simulink model "pkadai11"  (R2021b)
settings: Solver=VariableStepAuto  StartTime=0.0  StopTime=100  RelTol=1e-3
settings Model: Creator=is221042  LastModifiedBy=is221042

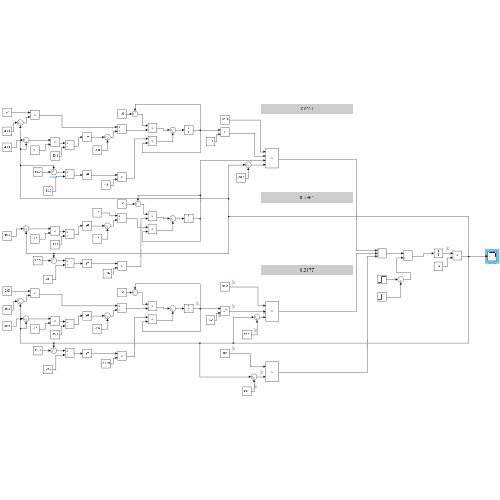
[thumbnail: Simulink's stored preview of the top-level diagram]
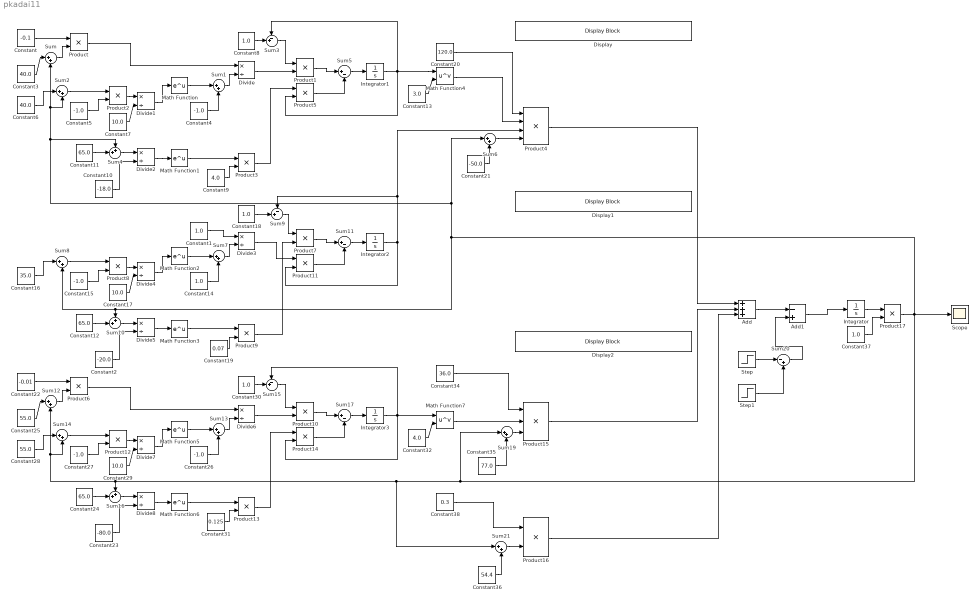
== system pkadai11 ==
  Add : Sum  Inputs=+++
  Add1 : Sum  Inputs=-+
  Constant : Constant  Value=-0.1
  Constant{1,8,14,18,30,37} (6 alike) : Constant  Value=1.0
  Constant10 : Constant  Value=-18.0
  Constant11 : Constant  Value=65.0
  Constant12 : Constant  Value=65.0
  Constant13 : Constant  Value=3.0
  Constant{4..5,15,26..27} (5 alike) : Constant  Value=-1.0
  Constant16 : Constant  Value=35.0
  Constant17 : Constant  Value=10.0
  Constant19 : Constant  Value=0.07
  Constant2 : Constant  Value=-20.0
  Constant20 : Constant  Value=120.0
  Constant21 : Constant  Value=-50.0
  Constant22 : Constant  Value=-0.01
  Constant23 : Constant  Value=-80.0
  Constant24 : Constant  Value=65.0
  Constant25 : Constant  Value=55.0
  Constant28 : Constant  Value=55.0
  Constant29 : Constant  Value=10.0
  Constant3 : Constant  Value=40.0
  Constant31 : Constant  Value=0.125
  Constant32 : Constant  Value=4.0
  Constant34 : Constant  Value=36.0
  Constant35 : Constant  Value=77.0
  Constant36 : Constant  Value=54.4
  Constant38 : Constant  Value=0.3
  Constant6 : Constant  Value=40.0
  Constant7 : Constant  Value=10.0
  Constant9 : Constant  Value=4.0
  Display : DisplayBlock  LabelPosition=Hide  Format=short  Transparency=1
  Display1 : DisplayBlock  LabelPosition=Hide  Format=short  Transparency=1
  Display2 : DisplayBlock  LabelPosition=Hide  Format=short  Transparency=1
  Divide{,1..8} (9 alike) : Product  Inputs=*/
  Integrator : Integrator  InitialCondition=-65.0
  Integrator1 : Integrator  InitialCondition=0.0529
  Integrator2 : Integrator  InitialCondition=0.4119
  Integrator3 : Integrator  InitialCondition=0.2668
  Math Function{,1..3,5..6} (6 alike) : Math  SaturateOnIntegerOverflow=on
  Math Function4 : Math  Operator=pow  SaturateOnIntegerOverflow=on
  Math Function7 : Math  Operator=pow  SaturateOnIntegerOverflow=on
  Product{,1..3,5..14,16..17} (16 alike) : Product
  Product15 : Product  Inputs=3
  Product4 : Product  Inputs=4
  Scope : Scope
  Step : Step  Time=4  After=5  SampleTime=0
  Step1 : Step  Time=2  After=5  SampleTime=0
  Sum{,1..2,6..8,12..14,19,21} (11 alike) : Sum  Inputs=|++
  Sum10 : Sum  Inputs=++|
  Sum11 : Sum  Inputs=|+-
  Sum15 : Sum  Inputs=-+|
  Sum16 : Sum  Inputs=++|
  Sum17 : Sum  Inputs=|+-
  Sum20 : Sum  Inputs=|-+
  Sum3 : Sum  Inputs=-+|
  Sum4 : Sum  Inputs=++|
  Sum5 : Sum  Inputs=|+-
  Sum9 : Sum  Inputs=-+|
  wires:
  Constant/1 -> Product/1
  Sum/1 -> Product/2
  Constant3/1 -> Sum/1
  Product/1 -> Divide/1
  Math Function/1 -> Sum1/1
  Sum1/1 -> Divide/2
  Constant4/1 -> Sum1/2
  Divide1/1 -> Math Function/1
  Sum2/1 -> Product2/1
  Product2/1 -> Divide1/1
  Constant5/1 -> Product2/2
  Constant6/1 -> Sum2/1
  Constant7/1 -> Divide1/2
  Constant8/1 -> Sum3/2
  Sum3/1 -> Product1/1
  Divide/1 -> Product1/2
  Sum4/1 -> Divide2/1
  Constant10/1 -> Divide2/2
  Constant11/1 -> Sum4/2
  Divide2/1 -> Math Function1/1
  Math Function1/1 -> Product3/1
  Constant9/1 -> Product3/2
  Integrator1/1 -> Product5/2, Math Function4/1, Sum3/1
  Product1/1 -> Sum5/1
  Product3/1 -> Product5/1
  Product5/1 -> Sum5/2
  Sum5/1 -> Integrator1/1
  Constant19/1 -> Product9/2
  Product11/1 -> Sum11/2
  Sum11/1 -> Integrator2/1
  Product7/1 -> Sum11/1
  Divide5/1 -> Math Function3/1
  Constant12/1 -> Sum10/2
  Math Function3/1 -> Product9/1
  Sum7/1 -> Divide3/2
  Constant15/1 -> Product8/2
  Constant17/1 -> Divide4/2
  Integrator2/1 -> Sum9/1, Product4/3, Product11/2
  Constant16/1 -> Sum8/1
  Constant18/1 -> Sum9/2
  Product8/1 -> Divide4/1
  Sum8/1 -> Product8/1
  Math Function2/1 -> Sum7/1
  Constant2/1 -> Divide5/2
  Sum10/1 -> Divide5/1
  Constant14/1 -> Sum7/2
  Sum9/1 -> Product7/1
  Divide4/1 -> Math Function2/1
  Constant1/1 -> Divide3/1
  Divide3/1 -> Product11/1
  Product9/1 -> Product7/2
  Constant13/1 -> Math Function4/2
  Constant20/1 -> Product4/1
  Math Function4/1 -> Product4/2
  Sum6/1 -> Product4/4
  Constant21/1 -> Sum6/2
  Product13/1 -> Product14/1
  Constant31/1 -> Product13/2
  Product14/1 -> Sum17/2
  Sum17/1 -> Integrator3/1
  Product10/1 -> Sum17/1
  Integrator3/1 -> Math Function7/1, Sum15/1, Product14/2
  Divide8/1 -> Math Function6/1
  Constant22/1 -> Product6/1
  Constant24/1 -> Sum16/2
  Constant25/1 -> Sum12/1
  Math Function6/1 -> Product13/1
  Sum13/1 -> Divide6/2
  Constant27/1 -> Product12/2
  Constant29/1 -> Divide7/2
  Product6/1 -> Divide6/1
  Divide6/1 -> Product10/2
  Constant28/1 -> Sum14/1
  Constant30/1 -> Sum15/2
  Product12/1 -> Divide7/1
  Sum12/1 -> Product6/2
  Math Function5/1 -> Sum13/1
  Constant23/1 -> Divide8/2
  Sum16/1 -> Divide8/1
  Constant26/1 -> Sum13/2
  Sum15/1 -> Product10/1
  Divide7/1 -> Math Function5/1
  Sum14/1 -> Product12/1
  Constant32/1 -> Math Function7/2
  Constant34/1 -> Product15/1
  Math Function7/1 -> Product15/2
  Sum19/1 -> Product15/3
  Constant35/1 -> Sum19/2
  Sum21/1 -> Product16/2
  Constant38/1 -> Product16/1
  Constant36/1 -> Sum21/2
  Integrator/1 -> Product17/1
  Product4/1 -> Add/1
  Product15/1 -> Add/2
  Product16/1 -> Add/3
  Add/1 -> Add1/1
  Add1/1 -> Integrator/1
  Constant37/1 -> Product17/2
  Product17/1 -> Sum8/2, Sum10/1, Sum6/1, Sum4/1, Sum2/2, Sum/2, Scope/1, Sum19/1, Sum21/1, Sum14/2, Sum12/2, Sum16/1
  Step/1 -> Sum20/1
  Sum20/1 -> Add1/2
  Step1/1 -> Sum20/2
